simulink model "Computed_Force"  (R2021b)
settings: Solver=VariableStepAuto  StartTime=0.0  StopTime=10.0  RelTol=1e-3
values from neighbouring files (symbols this model uses):
  Kp_I = 250    [datasheet.m]    (also in setup.m = 3000)
  R = tf([K*Lmax, K*R], [1 0])    [ElecTFanalysis.m]    (also in L.m = 3.7; LQRgen.m = 1; LQRsetup.m = 1; datasheet.m = 3.7)
  xD = d0/2    (= 0.00614)    [datasheet.m]    (also in setup.m)
libraries: MAGLEV_components x1, slpidlib x1
settings Model: Creator=dfigu  LastModifiedBy=dfigu

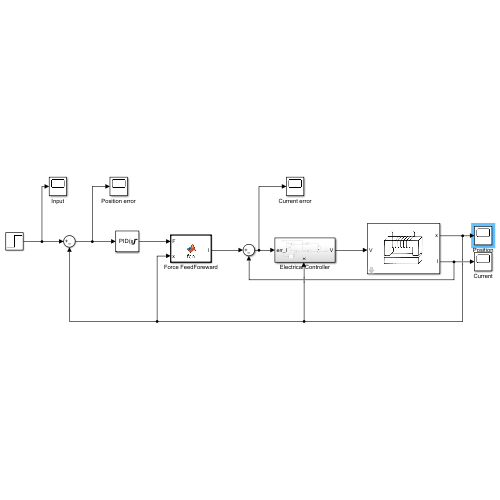
[thumbnail: Simulink's stored preview of the top-level diagram]
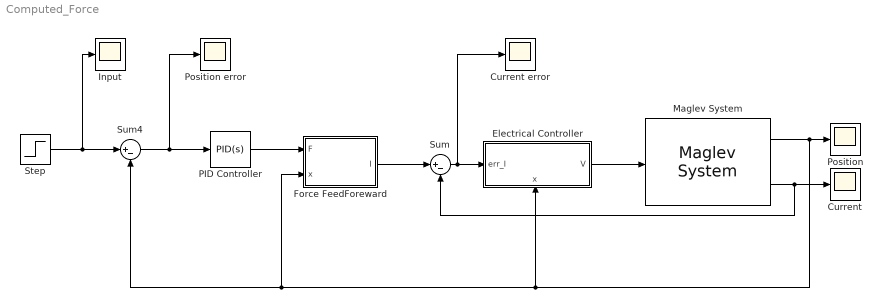
== system Computed_Force ==
  Current : Scope
  Current error : Scope
  Electrical Controller : Subsystem
      settings: PortSchema="{\"entries\":[{\"content\":{\"sides\":[{\"content\":{\"connectorIds\":[\"In1\"]},\"type\":\"ConnectorPlacement.EquallySpacedRectSide\",\"uuid\":\"2a1f29dc-395b-48bf-aa51-0c4dff6224aa\"},{\"content\":{\"connectorIds\":[\"Out1\"],\"side\":\"RIGHT\"},\"type\":\"ConnectorPlacement.EquallySpacedRectSide\",\"uuid\":\"9189c00b-28ea-4cda-9be7-751db9fa51ca\"},{\"content\":{\"connectorIds\":[],\"side\":\"TOP\"},\"type\":\"ConnectorPlacement.EquallySpacedRectSide\",\"uuid\":\"fd8e4d4f-79cd-4774-8370-9faf3c85e7eb\"},{\"content\":{\"connectorIds\":[\"In2\"],\"side\":\"BOTTOM\"},\"type\":\"ConnectorPlacement.EquallySpacedRectSide\",\"uuid\":\"84b0a39a-c969-4bb5-8f71-3c5847217c69\"}]},\"type\":\"ConnectorPlacement.EquallySpacedConnector\",\"uuid\":\"9aa78b26-320e-4dea-be36-119656051d58\"}],\"packageUris\":[\"http://schema.mathworks.com/mf0/Connector/R2020b\"],\"version\":\"1.0\"}"
  Force FeedForeward : MATLAB Function  TreatAsAtomicUnit=on
  Input : Scope
  Maglev System : MAGLEV_components/Maglev System
  PID Controller : slpidlib/PID Controller  Controller=PID  Form=Parallel  TimeDomain=Continuous-time  UseExternalTs=off  SampleTime=-1  IntegratorMethod=Forward Euler  FilterMethod=Forward Euler  ControllerParametersSource=internal  P=0.5  I=0.1  D=20  UseFilter=on  N=100  TunerSelectOption=Transfer Function Based (PID Tuner App)  InitialConditionSource=internal  InitialConditionForIntegrator=0  InitialConditionForFilter=0  DifferentiatorICPrevScaledInput=0  ExternalReset=none  TrackingMode=off  Kt=1  LimitOutput=on  SatLimitsSource=internal  UpperSaturationLimit=inf  LowerSaturationLimit=-inf  LinearizeAsGain=on  AntiWindupMode=back-calculation  Kb=100  POutMin=[]  POutMax=[]  IOutMin=[]  IOutMax=[]  DOutMin=[]  DOutMax=[]  NOutMin=[]  NOutMax=[]  SumOutMin=[]  SumOutMax=[]  SaturationOutMin=[]  SaturationOutMax=[]  PParamMin=[]  PParamMax=[]  IParamMin=[]  IParamMax=[]  DParamMin=[]  DParamMax=[]  NParamMin=[]  NParamMax=[]  KbParamMin=[]  KbParamMax=[]  KtParamMin=[]  KtParamMax=[]  KbOutMin=[]  KbOutMax=[]  KtOutMin=[]  KtOutMax=[]  IntegratorOutMin=[]  IntegratorOutMax=[]  FilterOutMin=[]  FilterOutMax=[]  SumI1OutMin=[]  SumI1OutMax=[]  SumI2OutMin=[]  SumI2OutMax=[]  SumI3OutMin=[]  SumI3OutMax=[]  SumI4OutMin=[]  SumI4OutMax=[]  SumDOutMin=[]  SumDOutMax=[]  DifferentiatorOutMin=[]  DifferentiatorOutMax=[]  FilterDiffOutCoefMin=[]  FilterDiffOutCoefMax=[]  ReciprocalOutMin=[]  ReciprocalOutMax=[]  SumDenOutMin=[]  SumDenOutMax=[]  SumNumOutMin=[]  SumNumOutMax=[]  DivideOutMin=[]  DivideOutMax=[]  UdiffTsProdOutMin=[]  UdiffTsProdOutMax=[]  NTsProdOutMin=[]  NTsProdOutMax=[]  UintegralTsProdOutMin=[]  UintegralTsProdOutMax=[]  UngainTsProdOutMin=[]  UngainTsProdOutMax=[]  IntegratorContinuousStateAttributes=''  IntegratorStateMustResolveToSignalObject=off  IntegratorRTWStateStorageClass=Auto  FilterContinuousStateAttributes=''  FilterStateMustResolveToSignalObject=off  FilterRTWStateStorageClass=Auto  ParallelPVariant=InternalParameters  IdealPVariant=Disabled  IVariant=InternalParameters  DVariant=InternalParameters  IntegratorVariant=Continuous  SatVariant=Enabled  AWVariant=BackCalculation  PCopyVariant=Disabled  TRVariant=Disabled  FdbkBlocksVariant=Forward  IdealPFdbkVariant=Disabled  SatFdbkVariant=Disabled  DerivativeFilterVariant=ContFilter  NVariant=InternalParameters  NCopyVariant=Disabled  FilterICVariant=InternalICsFilter  IntegratorICVariant=InternalICs  ExternalResetVariant=Disabled  TRSumVariant=Passthrough  SumFdbkVariant=Disabled  SumVariant=Sum_PID  TsampFilterVariant=InternalTs  TsampNgainVariant=Passthrough  TsampIntegralVariant=Passthrough  ExternalSaturationOutDataTypeStr=Inherit: Same as second input
  Position : Scope
  Position error : Scope
  Step : Step  Time=0  After=xD  SampleTime=0
  Sum : Sum  Inputs=|+-
  Sum4 : Sum  Inputs=|+-
  wires:
  Electrical Controller/1(V) -> Maglev System/1
  Maglev System/2 -> Current/1, Sum/2
  Sum/1 -> Electrical Controller/1(err_I), Current error/1
  Maglev System/1 -> Position/1, Electrical Controller/2(x), Sum4/2, Force FeedForeward/2(x)
  Force FeedForeward/1(I) -> Sum/1
  PID Controller/1 -> Force FeedForeward/1(F)
  Step/1 -> Input/1, Sum4/1
  Sum4/1 -> PID Controller/1, Position error/1

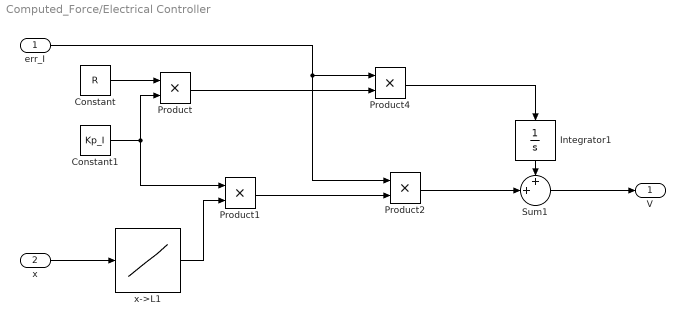
== system Computed_Force/Electrical Controller ==
  err_I : Inport
  x : Inport  Port=2
  Constant : Constant  Value=R
  Constant1 : Constant  Value=Kp_I
  Integrator1 : Integrator
  Product : Product
  Product1 : Product
  Product2 : Product  InputSameDT=on  RndMeth=Zero  SaturateOnIntegerOverflow=on  OutDataTypeStr=Inherit: Same as first input
  Product4 : Product  InputSameDT=on  RndMeth=Zero  SaturateOnIntegerOverflow=on  OutDataTypeStr=Inherit: Same as first input
  Sum1 : Sum  Inputs=++|  InputSameDT=on  SaturateOnIntegerOverflow=on  OutDataTypeStr=Inherit: Same as first input
  x->L1 : Lookup_n-D  NumberOfTableDimensions=1  BreakpointsForDimension1=[0,0.002,0.007,0.0096,0.011,0.0143,0.01445]  Table=[0.1086,0.114,0.129,0.148,0.165,0.250,0.350]  InternalRulePriority=Speed  RndMeth=Simplest  InputSameDT=on
  V : Outport
  wires:
  x/1 -> x->L1/1
  Constant/1 -> Product/1
  Constant1/1 -> Product/2, Product1/1
  x->L1/1 -> Product1/2
  Sum1/1 -> V/1
  err_I/1 -> Product2/1, Product4/1
  Product4/1 -> Integrator1/1
  Product/1 -> Product4/2
  Product1/1 -> Product2/2
  Product2/1 -> Sum1/2
  Integrator1/1 -> Sum1/1

== matlab function Computed_Force/Force FeedForeward ==
  data: F input; I output; x input
function I = fcn(F, x)
m = 0.83474;        %mass
N = 860;            %spires
Lb = 0.03;          %width
Pb = 0.03;          %depth
d0 = 0.01228;       %delta0
u0 = 4*pi*10^(-7);  %permeabilità vuoto
cr = 700;           %coefficiente magnetismo ferro
Lfe = 0.2781;       %Lunghezza circuito ferro

As = Lb*Pb;
k = u0*As*(N^2);
I = sqrt(abs((m*9.81+F)*(Lfe/cr+2*(d0-x))^2)/k);
